simulink model "Problem_3"  (R2022b)
settings: Solver=VariableStepAuto  StartTime=0.0  StopTime=10.0  RelTol=1e-3
values from neighbouring files (symbols this model uses):
  bj = 10    [problm_3.m]
  bp = 100    [problm_3.m]
  g = 9.81    [problm_3.m]
  kr = 400    [problm_3.m]
  mj = 60    [problm_3.m]
  mp = 10    [problm_3.m]
settings Model: Creator=adnzw  LastModifiedBy=adnzw

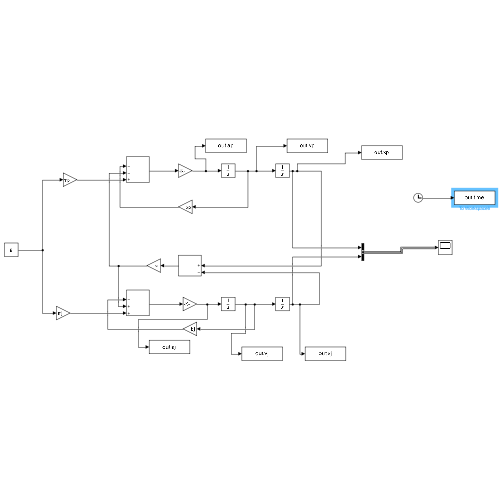
[thumbnail: Simulink's stored preview of the top-level diagram]
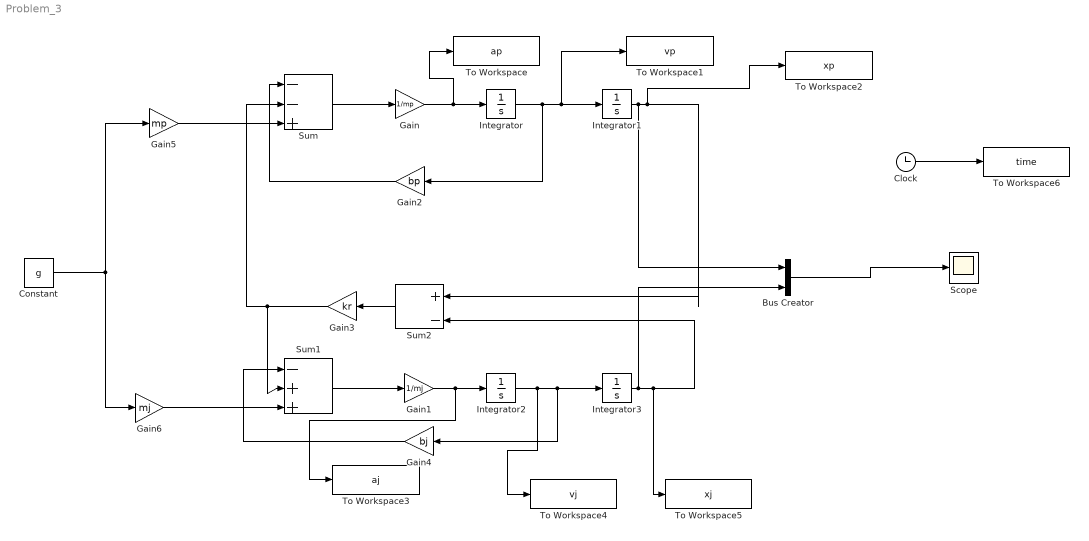
== system Problem_3 ==
  Bus Creator : BusCreator  Inputs=2
  Clock : Clock
  Constant : Constant  Value=g
  Gain : Gain  Gain=1/mp
  Gain1 : Gain  Gain=1/mj
  Gain2 : Gain  Gain=bp
  Gain3 : Gain  Gain=kr
  Gain4 : Gain  Gain=bj
  Gain5 : Gain  Gain=mp
  Gain6 : Gain  Gain=mj
  Integrator{,1..3} (4 alike) : Integrator
  Scope : Scope
  Sum : Sum  Inputs=|--+
  Sum1 : Sum  Inputs=|-++
  Sum2 : Sum  Inputs=|+-
  To Workspace : ToWorkspace  VariableName=ap  SaveFormat=Timeseries  SampleTime=-1
  To Workspace1 : ToWorkspace  VariableName=vp  SaveFormat=Timeseries  SampleTime=-1
  To Workspace2 : ToWorkspace  VariableName=xp  SaveFormat=Timeseries  SampleTime=-1
  To Workspace3 : ToWorkspace  VariableName=aj  SaveFormat=Timeseries  SampleTime=-1
  To Workspace4 : ToWorkspace  VariableName=vj  SaveFormat=Timeseries  SampleTime=-1
  To Workspace5 : ToWorkspace  VariableName=xj  SaveFormat=Timeseries  SampleTime=-1
  To Workspace6 : ToWorkspace  VariableName=time  SaveFormat=Timeseries  SampleTime=-1
  wires:
  Sum/1 -> Gain/1
  Gain/1 -> To Workspace/1, Integrator/1
  Integrator/1 -> Gain2/1, To Workspace1/1, Integrator1/1
  Gain1/1 -> To Workspace3/1, Integrator2/1
  Integrator2/1 -> To Workspace4/1, Gain4/1, Integrator3/1
  Gain2/1 -> Sum/1
  Sum1/1 -> Gain1/1
  Integrator1/1 -> Bus Creator/1, To Workspace2/1, Sum2/1
  Integrator3/1 -> Bus Creator/2, To Workspace5/1, Sum2/2
  Sum2/1 -> Gain3/1
  Gain4/1 -> Sum1/1
  Constant/1 -> Gain5/1, Gain6/1
  Bus Creator/1 -> Scope/1
  Gain3/1 -> Sum1/2, Sum/2
  Gain5/1 -> Sum/3
  Gain6/1 -> Sum1/3
  Clock/1 -> To Workspace6/1
